simulink library "SIXOSEM_F_WD_DC_MASTER"  (Simulink 8.0)
settings: Solver=ode45  StartTime=0.0  StopTime=10.0  RelTol=1e-3
libraries: cdsFilt x6, cdsEpicsIn x2
settings Model: Creator=controls  LastModifiedBy=controls

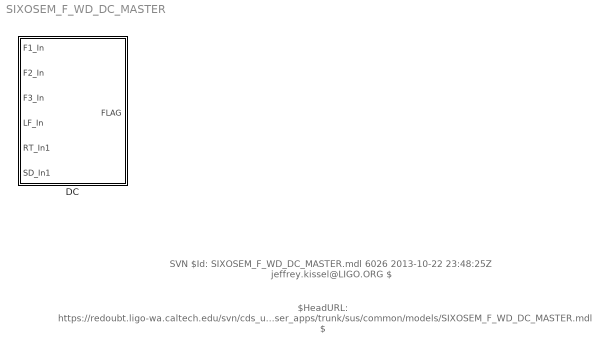
== system SIXOSEM_F_WD_DC_MASTER ==
  note: $HeadURL: https://redoubt.ligo-wa.caltech.edu/svn/cds_user_apps/trunk/sus/common/models/SIXOSEM_F_WD_DC_MASTER.mdl $
  note: SVN $Id: SIXOSEM_F_WD_DC_MASTER.mdl 6026 2013-10-22 23:48:25Z jeffrey.kissel@LIGO.ORG $
  DC : Subsystem

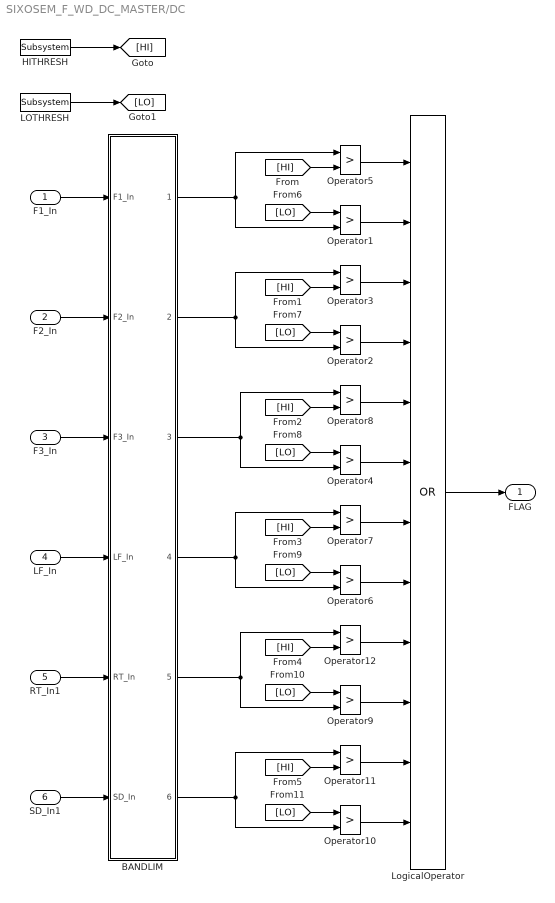
== system SIXOSEM_F_WD_DC_MASTER/DC ==
  F1_In : Inport
  F2_In : Inport  Port=2
  F3_In : Inport  Port=3
  LF_In : Inport  Port=4
  RT_In1 : Inport  Port=5
  SD_In1 : Inport  Port=6
  BANDLIM : Subsystem
  HITHRESH : cdsEpicsIn/Subsystem  Tag=cdsEpicsIn  Description=|  SystemSampleTime=-1
      | Purpose:                                                                              
      | Create an EPICS input channel connection to the FE realtime controls.                 
      |                                                                                       
      | Operation:                                                                            
      | Outputs value from an EPICS ai record. Value is floating point with a precision of 3..
      |                                                                                       
      | Usage:                                                                                
      | Name the part with the desired EPICS channel name.
      settings: AttributesFormatString=%<Tag>
  LOTHRESH : cdsEpicsIn/Subsystem  Tag=cdsEpicsIn  Description=|  SystemSampleTime=-1
      | Purpose:                                                                              
      | Create an EPICS input channel connection to the FE realtime controls.                 
      |                                                                                       
      | Operation:                                                                            
      | Outputs value from an EPICS ai record. Value is floating point with a precision of 3..
      |                                                                                       
      | Usage:                                                                                
      | Name the part with the desired EPICS channel name.
      settings: AttributesFormatString=%<Tag>
  LogicalOperator : Logic  Operator=OR  Inputs=12  AllPortsSameDT=off  OutDataTypeStr=boolean
  Operator{1..12} (12 alike) : RelationalOperator  Operator=>  OutDataTypeStr=boolean
  FLAG : Outport
  wires:
  SD_In1/1 -> BANDLIM/6(SD_In)
  RT_In1/1 -> BANDLIM/5(RT_In)
  LF_In/1 -> BANDLIM/4(LF_In)
  F3_In/1 -> BANDLIM/3(F3_In)
  F2_In/1 -> BANDLIM/2(F2_In)
  F1_In/1 -> BANDLIM/1(F1_In)
  LogicalOperator/1 -> FLAG/1
  BANDLIM/1(F1_Out) -> Operator1/2, Operator5/1
  Operator5/1 -> LogicalOperator/1
  Operator1/1 -> LogicalOperator/2
  Operator3/1 -> LogicalOperator/3
  Operator2/1 -> LogicalOperator/4
  BANDLIM/2(F2_Out) -> Operator2/2, Operator3/1
  Operator8/1 -> LogicalOperator/5
  Operator4/1 -> LogicalOperator/6
  Operator7/1 -> LogicalOperator/7
  Operator6/1 -> LogicalOperator/8
  BANDLIM/4(LF_Out) -> Operator6/2, Operator7/1
  BANDLIM/3(F3_Out) -> Operator4/2, Operator8/1
  Operator12/1 -> LogicalOperator/9
  Operator9/1 -> LogicalOperator/10
  Operator11/1 -> LogicalOperator/11
  Operator10/1 -> LogicalOperator/12
  BANDLIM/6(SD_Out) -> Operator10/2, Operator11/1
  BANDLIM/5(RT_Out) -> Operator9/2, Operator12/1
  HITHRESH/1 -> [HI]
  LOTHRESH/1 -> [LO]
  [HI] -> Operator5/2
  [HI] -> Operator3/2
  [HI] -> Operator8/2
  [HI] -> Operator7/2
  [HI] -> Operator12/2
  [HI] -> Operator11/2
  [LO] -> Operator1/1
  [LO] -> Operator2/1
  [LO] -> Operator4/1
  [LO] -> Operator6/1
  [LO] -> Operator9/1
  [LO] -> Operator10/1

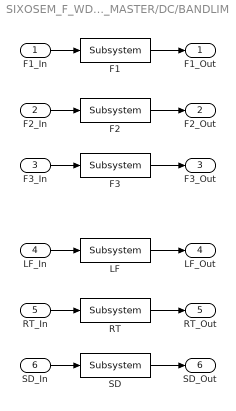
== system SIXOSEM_F_WD_DC_MASTER/DC/BANDLIM ==
  F1_In : Inport
  F2_In : Inport  Port=2
  F3_In : Inport  Port=3
  LF_In : Inport  Port=4
  RT_In : Inport  Port=5
  SD_In : Inport  Port=6
  F1 : cdsFilt/Subsystem  Tag=cdsFilt  Description=|  SystemSampleTime=-1
      | Purpose:                                                                                                                                                                                                                                  
      | Standard CDS IIR filter module.                                                                                                                                                                                                           
      |                                                                                                                                                                                                                                           
      | Operation:                                                                                                                                                                                                                                
      | Consists of 10 second order section IIR filters, plus a ramped gain stage. In FE code, also provides pre-defined test points and excitation channel inputs. The filter coefficients are defined in the LIGO system using the 'foton' tool.
      |                                                                                                                                                                                                                                           
      | Usage:                                                                                                                                                                                                                                    
      | Name the part with the desired filter module name.
      settings: AttributesFormatString=%<Tag>
  F2 : cdsFilt/Subsystem  Tag=cdsFilt  Description=|  SystemSampleTime=-1
      | Purpose:                                                                                                                                                                                                                                  
      | Standard CDS IIR filter module.                                                                                                                                                                                                           
      |                                                                                                                                                                                                                                           
      | Operation:                                                                                                                                                                                                                                
      | Consists of 10 second order section IIR filters, plus a ramped gain stage. In FE code, also provides pre-defined test points and excitation channel inputs. The filter coefficients are defined in the LIGO system using the 'foton' tool.
      |                                                                                                                                                                                                                                           
      | Usage:                                                                                                                                                                                                                                    
      | Name the part with the desired filter module name.
      settings: AttributesFormatString=%<Tag>
  F3 : cdsFilt/Subsystem  Tag=cdsFilt  Description=|  SystemSampleTime=-1
      | Purpose:                                                                                                                                                                                                                                  
      | Standard CDS IIR filter module.                                                                                                                                                                                                           
      |                                                                                                                                                                                                                                           
      | Operation:                                                                                                                                                                                                                                
      | Consists of 10 second order section IIR filters, plus a ramped gain stage. In FE code, also provides pre-defined test points and excitation channel inputs. The filter coefficients are defined in the LIGO system using the 'foton' tool.
      |                                                                                                                                                                                                                                           
      | Usage:                                                                                                                                                                                                                                    
      | Name the part with the desired filter module name.
      settings: AttributesFormatString=%<Tag>
  LF : cdsFilt/Subsystem  Tag=cdsFilt  Description=|  SystemSampleTime=-1
      | Purpose:                                                                                                                                                                                                                                  
      | Standard CDS IIR filter module.                                                                                                                                                                                                           
      |                                                                                                                                                                                                                                           
      | Operation:                                                                                                                                                                                                                                
      | Consists of 10 second order section IIR filters, plus a ramped gain stage. In FE code, also provides pre-defined test points and excitation channel inputs. The filter coefficients are defined in the LIGO system using the 'foton' tool.
      |                                                                                                                                                                                                                                           
      | Usage:                                                                                                                                                                                                                                    
      | Name the part with the desired filter module name.
      settings: AttributesFormatString=%<Tag>
  RT : cdsFilt/Subsystem  Tag=cdsFilt  Description=|  SystemSampleTime=-1
      | Purpose:                                                                                                                                                                                                                                  
      | Standard CDS IIR filter module.                                                                                                                                                                                                           
      |                                                                                                                                                                                                                                           
      | Operation:                                                                                                                                                                                                                                
      | Consists of 10 second order section IIR filters, plus a ramped gain stage. In FE code, also provides pre-defined test points and excitation channel inputs. The filter coefficients are defined in the LIGO system using the 'foton' tool.
      |                                                                                                                                                                                                                                           
      | Usage:                                                                                                                                                                                                                                    
      | Name the part with the desired filter module name.
      settings: AttributesFormatString=%<Tag>
  SD : cdsFilt/Subsystem  Tag=cdsFilt  Description=|  SystemSampleTime=-1
      | Purpose:                                                                                                                                                                                                                                  
      | Standard CDS IIR filter module.                                                                                                                                                                                                           
      |                                                                                                                                                                                                                                           
      | Operation:                                                                                                                                                                                                                                
      | Consists of 10 second order section IIR filters, plus a ramped gain stage. In FE code, also provides pre-defined test points and excitation channel inputs. The filter coefficients are defined in the LIGO system using the 'foton' tool.
      |                                                                                                                                                                                                                                           
      | Usage:                                                                                                                                                                                                                                    
      | Name the part with the desired filter module name.
      settings: AttributesFormatString=%<Tag>
  F1_Out : Outport
  F2_Out : Outport  Port=2
  F3_Out : Outport  Port=3
  LF_Out : Outport  Port=4
  RT_Out : Outport  Port=5
  SD_Out : Outport  Port=6
  wires:
  F1/1 -> F1_Out/1
  F2/1 -> F2_Out/1
  F3/1 -> F3_Out/1
  F1_In/1 -> F1/1
  F2_In/1 -> F2/1
  F3_In/1 -> F3/1
  LF/1 -> LF_Out/1
  RT/1 -> RT_Out/1
  SD/1 -> SD_Out/1
  LF_In/1 -> LF/1
  RT_In/1 -> RT/1
  SD_In/1 -> SD/1
